simulink model "Probar_Colison"  (R2024b)
settings: Solver=VariableStepAuto  StartTime=0.0  StopTime=inf  RelTol=1e-3
libraries: simulink x1
settings Model: Creator=Chenfu  LastModifiedBy=Chenfu

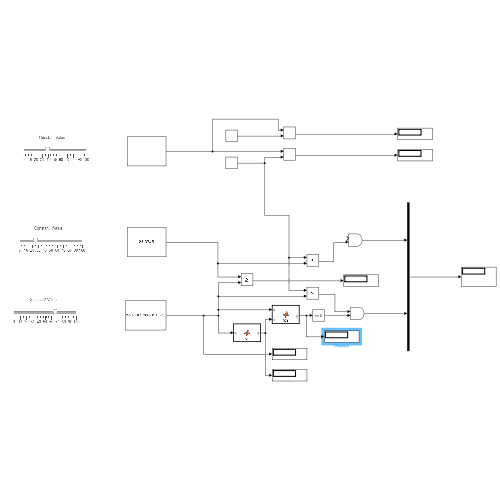
[thumbnail: Simulink's stored preview of the top-level diagram]
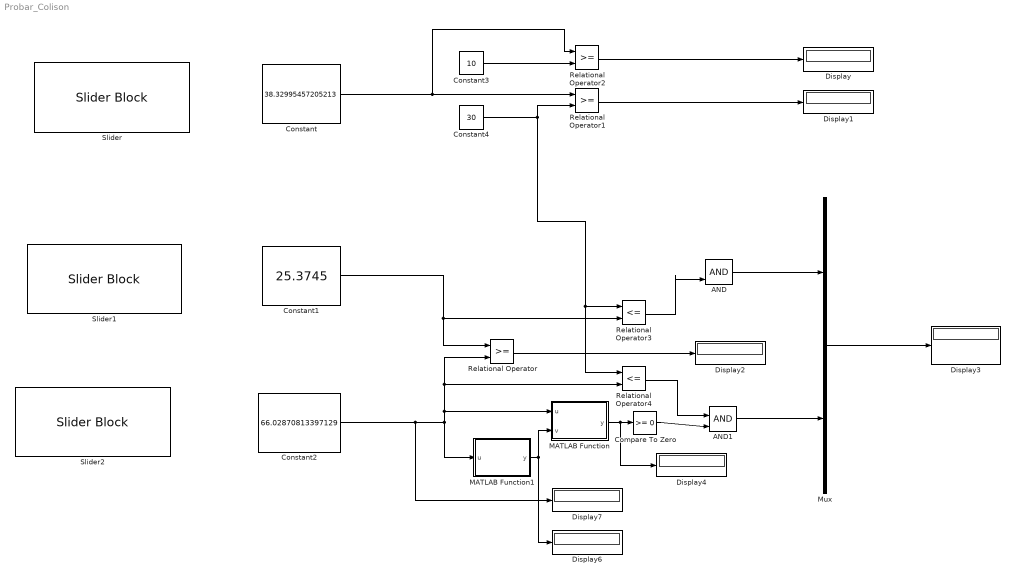
== system Probar_Colison ==
  AND : Logic  IconShape=distinctive  AllPortsSameDT=off  OutDataTypeStr=boolean
  AND1 : Logic  IconShape=distinctive  AllPortsSameDT=off  OutDataTypeStr=boolean
  Compare To Zero : simulink/Logic and Bit Operations/Compare To Zero  relop=>=  OutDataTypeStr=boolean
  Constant : Constant  Value=38.32995457205213
  Constant1 : Constant  Value=25.3745
  Constant2 : Constant  Value=66.02870813397129
  Constant3 : Constant  Value=10
  Constant4 : Constant  Value=30
  Display{,1..4,6..7} (7 alike) : Display
  MATLAB Function : MATLAB Function  TreatAsAtomicUnit=on
  MATLAB Function1 : MATLAB Function  TreatAsAtomicUnit=on
  Mux : Mux  Inputs=2
  Relational Operator : RelationalOperator  OutDataTypeStr=boolean  RndMeth=Simplest  InputSameDT=off
  Relational Operator1 : RelationalOperator  OutDataTypeStr=boolean  RndMeth=Simplest  InputSameDT=off
  Relational Operator2 : RelationalOperator  OutDataTypeStr=boolean  RndMeth=Simplest  InputSameDT=off
  Relational Operator3 : RelationalOperator  Operator=<=  OutDataTypeStr=boolean  RndMeth=Simplest  InputSameDT=off
  Relational Operator4 : RelationalOperator  Operator=<=  OutDataTypeStr=boolean  RndMeth=Simplest  InputSameDT=off
  Slider : SliderBlock
  Slider1 : SliderBlock
  Slider2 : SliderBlock
  wires:
  Mux/1 -> Display3/1
  Relational Operator/1 -> Display2/1
  Constant/1 -> Relational Operator1/1, Relational Operator2/1
  Constant1/1 -> Relational Operator/1, Relational Operator3/2
  Relational Operator1/1 -> Display1/1
  Constant4/1 -> Relational Operator1/2, Relational Operator4/1, Relational Operator3/1
  Relational Operator2/1 -> Display/1
  Constant3/1 -> Relational Operator2/2
  AND/1 -> Mux/1
  AND1/1 -> Mux/2
  Relational Operator3/1 -> AND/2
  Relational Operator4/1 -> AND1/1
  MATLAB Function1/1(y) -> MATLAB Function/2(v), Display6/1
  Compare To Zero/1 -> AND1/2
  MATLAB Function/1(y) -> Display4/1, Compare To Zero/1
  Constant2/1 -> Display7/1, MATLAB Function1/1(u), MATLAB Function/1(u), Relational Operator/2, Relational Operator4/2

== matlab function Probar_Colison/MATLAB Function ==
  data: u input; y output; v input
function y = fcn(u,v)

y = u-v;

== matlab function Probar_Colison/MATLAB Function1 ==
  data: u input; y output
function y = fcn(u)

pause(1);

y = u;
